simulink model "LLC_Resonant_Converter_v1"  (R2024b)
settings: Solver=FixedStepDiscrete  StartTime=0.0  StopTime=0.3  FixedStep=Ts_Power  MaxStep=1e-7  RelTol=1e-4  EnableMultiTasking=on
PreLoadFcn:
  | LLC_Resonant_Converter_v1_data
values from neighbouring files (symbols this model uses):
  Co = 150e-6    (= 0.00015)    [LLC_Resonant_Converter_v1_data.m]    (also in OBC_v1_data.m)
  Cr = 75e-9    (= 7.5e-08)    [LLC_Resonant_Converter_v1_data.m]    (also in OBC_v1_data.m)
  fs_LCC_max = 250e3    (= 250000)    [LLC_Resonant_Converter_v1_data.m]    (also in OBC_v1_data.m = 300000)
  fs_LCC_min = 120e3    (= 120000)    [LLC_Resonant_Converter_v1_data.m]    (also in OBC_v1_data.m)
  Ki_LLC = 150e3    (= 150000)    [LLC_Resonant_Converter_v1_data.m]    (also in OBC_v1_data.m)
  Kp_LLC = 100    [LLC_Resonant_Converter_v1_data.m]    (also in OBC_v1_data.m = 25)
  Lm = 150e-6    (= 0.00015)    [LLC_Resonant_Converter_v1_data.m]    (also in OBC_v1_data.m)
  Lr = 25e-6    (= 2.5e-05)    [LLC_Resonant_Converter_v1_data.m]    (also in OBC_v1_data.m)
  Np = 10    [LLC_Resonant_Converter_v1_data.m]    (also in OBC_v1_data.m)
  Ns = 12    [LLC_Resonant_Converter_v1_data.m]    (also in OBC_v1_data.m)
  Po_nom = 7.2e3    (= 7200)    [LLC_Resonant_Converter_v1_data.m]    (also in OBC_v1_data.m)
  Ts_Control = 10e-6    (= 1e-05)    [LLC_Resonant_Converter_v1_data.m]    (also in OBC_v1_data.m; Totem_Pole_PFC_v1_data.m)
  Ts_Power = 50e-9    (= 5e-08)    [LLC_Resonant_Converter_v1_data.m]    (also in OBC_v1_data.m; Totem_Pole_PFC_v1_data.m)
  Vdc_in = 400    [LLC_Resonant_Converter_v1_data.m]    (also in OBC_v1_data.m)
  Vo_nom = 400    [LLC_Resonant_Converter_v1_data.m]    (also in OBC_v1_data.m)
undefined symbols (not defined in the file or in its folder): DiscIntNeverNeededParam
libraries: spsSeriesRLCBranchLib x5, spsDiodeLib x4, MyLibrary x4, spsMeanLib x3, spsCurrentMeasurementLib x3, spsVoltageMeasurementLib x3, spsOnDelayLib x2, spsDCVoltageSourceLib x1, spsIdealSwitchLib x1, spsLinearTransformerLib x1, spspowerguiLib x1
settings Model: SimulationMode=accelerator  Creator=The MathWorks, Inc.  LastModifiedBy=santh
settings SolverCC: AlgebraicLoopSolver=TrustRegion  SolverResetMethod=Robust
settings DataIOCC: SaveOutput=off  SignalLogging=off  DSMLogging=off  SaveTime=off  ReturnWorkspaceOutputs=off
settings OptimizationCC: LifeSpan=inf
settings DebuggingCC: UnconnectedInputMsg=warning  UnconnectedOutputMsg=warning  UnconnectedLineMsg=warning  SFUnexpectedBacktrackingDiag=warning  SFNoUnconditionalDefaultTransitionDiag=warning  SFExecutionAtInitializationDiag=none  ArithmeticOperatorsInVariantConditions=warning
settings ModelReferenceCC: EnableRefExpFcnMdlSchedulingChecks=on
settings SFSimCC: SimUseLocalCustomCode=off  CustomCodeUndefinedFunction=UseInterfaceOnly
settings RTWCC: RTWUseLocalCustomCode=off  GPUComputeCapability=3.5  DLArmComputeVersion=19.05
settings CodeAppCC: StateflowObjectComments=on
settings GRTTargetCC: TargetLangStandard=C89/C90 (ANSI)
settings ConfigComp: CovMetricSettings=dw  CovSaveCumulativeToWorkspaceVar=on  CovSaveSingleToWorkspaceVar=on  CovExternalEMLEnable=off
settings SimscapeCC: SimscapeNormalizeSystem=off  SimscapeNominalValues={1, 'bar'; 1, 'cm^3/s'; 1, 'bar*kg/s'; 1, 'kJ/kg'; 1, 'kW'; }

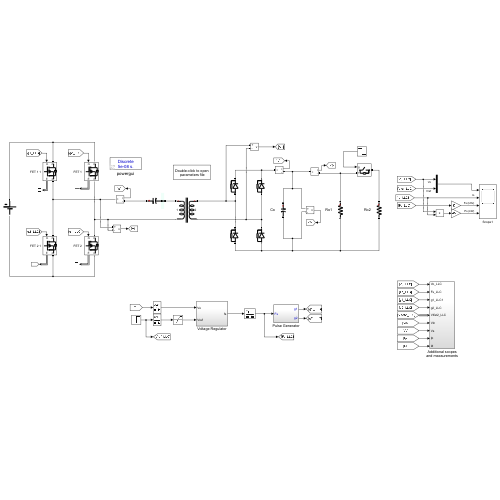
[thumbnail: Simulink's stored preview of the top-level diagram]
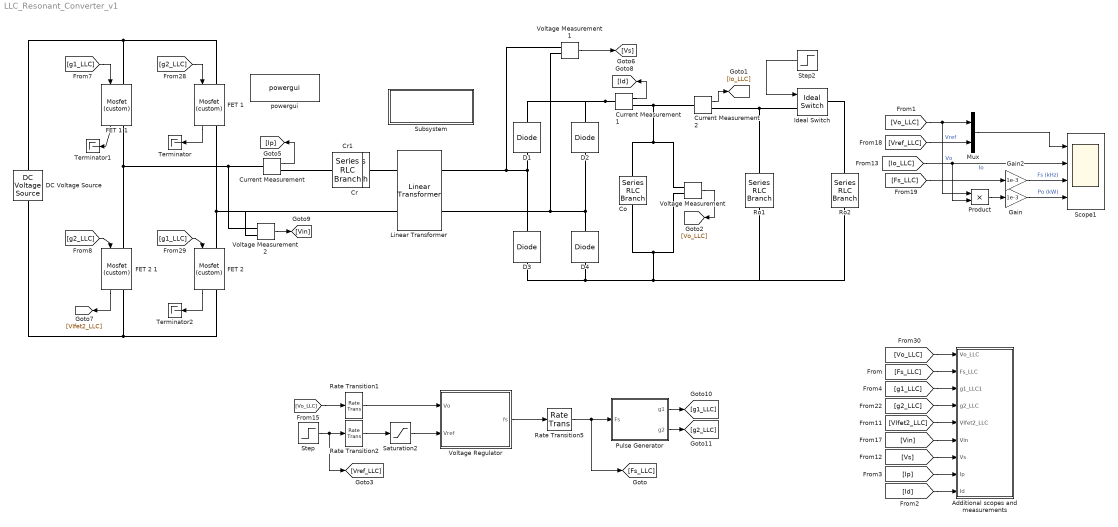
== system LLC_Resonant_Converter_v1 ==
  Additional scopes and measurements : Subsystem
  Co : spsSeriesRLCBranchLib/Series RLC Branch  LConnTagsString=__new0  RConnTagsString=__new0  BranchType=C  Resistance=1e-4  Inductance=200e-6  SetiL0=off  InitialCurrent=0  Capacitance=Co  Setx0=on  InitialVoltage=350  Measurements=None
  Cr : spsSeriesRLCBranchLib/Series RLC Branch  LConnTagsString=__new0  RConnTagsString=__new0  BranchType=C  Resistance=1e-4  Inductance=200e-6  SetiL0=off  InitialCurrent=0  Capacitance=Cr  Setx0=off  InitialVoltage=40  Measurements=None
  Cr1 : spsSeriesRLCBranchLib/Series RLC Branch  LConnTagsString=__new0  RConnTagsString=__new0  BranchType=C  Resistance=1e-4  Inductance=200e-6  SetiL0=off  InitialCurrent=0  Capacitance=Cr  Setx0=off  InitialVoltage=40  Measurements=None
  Current Measurement : spsCurrentMeasurementLib/Current Measurement  PhasorSimulation=off  OutputType=Complex  PSBequivalent=0
  Current Measurement1 : spsCurrentMeasurementLib/Current Measurement  PhasorSimulation=off  OutputType=Complex  PSBequivalent=0
  Current Measurement2 : spsCurrentMeasurementLib/Current Measurement  PhasorSimulation=off  OutputType=Complex  PSBequivalent=0
  D{1..4} (4 alike) : spsDiodeLib/Diode  Ron=Ron_Diode  Lon=0  Vf=Vf  IC=0  UseSnubber=off  Rs=1e6  Cs=inf  Measurements=off
  DC Voltage Source : spsDCVoltageSourceLib/DC Voltage Source  Amplitude=Vdc_in  Measurements=None
  "FET 1 " : MyLibrary/Mosfet (custom)  Ron=Ron_FET  Lon=0  Rd=Ron_Diode  Vfd=Vf  IC=0  Rs=1e6  Cs=inf  Measurements=on
  FET 1 1 : MyLibrary/Mosfet (custom)  Ron=Ron_FET  Lon=0  Rd=Ron_Diode  Vfd=Vf  IC=0  Rs=1e6  Cs=inf  Measurements=on
  "FET 2 " : MyLibrary/Mosfet (custom)  Ron=Ron_FET  Lon=0  Rd=Ron_Diode  Vfd=Vf  IC=0  Rs=1e6  Cs=inf  Measurements=on
  FET 2 1 : MyLibrary/Mosfet (custom)  Ron=Ron_FET  Lon=0  Rd=Ron_Diode  Vfd=Vf  IC=0  Rs=1e6  Cs=inf  Measurements=on
  Gain : Gain  Gain=1e-3
  Gain2 : Gain  Gain=1e-3
  Ideal Switch : spsIdealSwitchLib/Ideal Switch  Ron=0.001  Lon=0  IC=1  Rs=1e5  Cs=inf  Measurements=off
  Linear Transformer : spsLinearTransformerLib/Linear Transformer  UNITS=SI  NominalPower=[ 7000 100e3 ]  winding1="[Np   1e-2 Lr]"  winding2="[Ns  1e-2  1e-8 ]"  ThreeWindings=off  winding3=[3.15e+05 0.7938 0.084225]  RmLm=[1e4 Lm]  Measurements=None  DataType=on
  Mux : Mux  Inputs=2
  Product : Product
  Pulse Generator : Subsystem
  Rate Transition1 : RateTransition  OutPortSampleTime=Ts_Control
  Rate Transition2 : RateTransition  OutPortSampleTime=Ts_Control
  Rate Transition5 : RateTransition  InitialCondition=fs_LCC_min  OutPortSampleTime=Ts_Power
  Ro1 : spsSeriesRLCBranchLib/Series RLC Branch  LConnTagsString=__new0  RConnTagsString=__new0  BranchType=R  Resistance=Vo_nom^2/(0.1*Po_nom)  Inductance=200e-6  SetiL0=off  InitialCurrent=0  Capacitance=400e-6  Setx0=off  InitialVoltage=0  Measurements=None
  Ro2 : spsSeriesRLCBranchLib/Series RLC Branch  LConnTagsString=__new0  RConnTagsString=__new0  BranchType=R  Resistance=Vo_nom^2/(0.9*Po_nom)  Inductance=200e-6  SetiL0=off  InitialCurrent=0  Capacitance=400e-6  Setx0=off  InitialVoltage=0  Measurements=None
  Saturation2 : Saturate  UpperLimit=450  LowerLimit=275
  Scope1 : Scope  NumInputPorts=4
  Step : Step  Time=0.1  Before=350  After=400  SampleTime=Ts_Power
  Step2 : Step  Time=0.2  Before=1  After=0  SampleTime=Ts_Power
  Subsystem : Subsystem
      settings: OpenFcn=edit('LLC_Resonant_Converter_v1_data');
      mask Display: disp('Double-click to open\n parameters file');
  Terminator : Terminator
  Terminator1 : Terminator
  Terminator2 : Terminator
  Voltage Measurement : spsVoltageMeasurementLib/Voltage Measurement  PhasorSimulation=off  OutputType=Complex  PSBequivalent=0
  Voltage Measurement1 : spsVoltageMeasurementLib/Voltage Measurement  PhasorSimulation=off  OutputType=Complex  PSBequivalent=0
  Voltage Measurement2 : spsVoltageMeasurementLib/Voltage Measurement  PhasorSimulation=off  OutputType=Complex  PSBequivalent=0
  Voltage Regulator : Subsystem
  powergui : spspowerguiLib/powergui  Priority=1  SimulationMode=Discrete  SampleTime=Ts_Power  frequency=60  Iterations=50  frequencyindice=0  Pbase=100e6  ErrMax=1e-4  UnitsV=kV  UnitsW=MW  buscounter=0  FunctionMessages=off  echomessages=off  EnableUseOfTLC=off  CurrentSourceSwitches=off  DisableSnubberDevices=off  DisableRonSwitches=off  DisableVfSwitches=off  DisplayEquations=off  AutomaticDiscreteSolvers=off  SolverType=Tustin/Backward Euler (TBE)  Interpol=off  ExternalGateDelay=off  methode=off  Ts=100  x0status=blocks  SPID=on  SwTol=0  HookPort=off  NonlinearTolerance=1e-4  nMaxIteration=100  ContinueOnMaxIteration=off  RestoreLinks=warning  ResistiveCurrentMeasurement=off  Frange=[0:2:500]  Ylog=off  Xlog=on  ShowGrid=off  save=off  variable=ZData  structure=0  ZoomFFT=off  StartTime=0.0  cycles=1  DisplayStyle=1  fundamental=60  FreqAxis=off  MaxFrequency=1000  frequencyindicesteady=1  RmsSteady=1  display=off
  wires:
  [g1_LLC] -> "FET 2 "/1
  Current Measurement/1 -> [Ip]
  Voltage Measurement/1 -> [Vo_LLC]
  Current Measurement1/1 -> [Id]
  [Vo_LLC] -> Rate Transition1/1
  Pulse Generator/1(g1) -> [g1_LLC]
  Pulse Generator/2(g2) -> [g2_LLC]
  Current Measurement2/1 -> [Io_LLC]
  "FET 1 "/1 -> Terminator/1
  Rate Transition2/1 -> Saturation2/1
  Saturation2/1 -> Voltage Regulator/2(Vref)
  Step/1 -> [Vref_LLC], Rate Transition2/1
  Rate Transition1/1 -> Voltage Regulator/1(Vo)
  Step2/1 -> Ideal Switch/1
  [g2_LLC] -> "FET 1 "/1
  "FET 2 "/1 -> Terminator2/1
  Gain2/1 -> Scope1/3  "Fs (kHz)"
  [Vref_LLC] -> Mux/2  "Vref"
  Product/1 -> Gain/1
  [Io_LLC] -> Product/2, Scope1/2  "Io"
  [Vo_LLC] -> Product/1, Mux/1  "Vo"
  [Fs_LLC] -> Gain2/1
  Gain/1 -> Scope1/4  "Po (kW)"
  Voltage Measurement1/1 -> [Vs]
  Voltage Measurement2/1 -> [Vin]
  Rate Transition5/1 -> [Fs_LLC], Pulse Generator/1(Fs)
  FET 2 1/1 -> [VIfet2_LLC]
  [g1_LLC] -> FET 1 1/1
  FET 1 1/1 -> Terminator1/1
  [g2_LLC] -> FET 2 1/1
  Voltage Regulator/1(fs) -> Rate Transition5/1
  [Vo_LLC] -> Additional scopes and measurements/1(Vo_LLC)
  [Fs_LLC] -> Additional scopes and measurements/2(Fs_LLC)
  [g2_LLC] -> Additional scopes and measurements/4(g2_LLC)
  [Vs] -> Additional scopes and measurements/7(Vs)
  [Vin] -> Additional scopes and measurements/6(Vin)
  [Id] -> Additional scopes and measurements/9(Id)
  [Ip] -> Additional scopes and measurements/8(Ip)
  Mux/1 -> Scope1/1
  [g1_LLC] -> Additional scopes and measurements/3(g1_LLC1)
  [VIfet2_LLC] -> Additional scopes and measurements/5(VIfet2_LLC)
  connections:
  Co/RConn1 -- Voltage Measurement/LConn2 -- Ro2/RConn1 -- Ro1/RConn1 -- D3/LConn1 -- D4/LConn1
  Linear Transformer/RConn1 -- D3/RConn1 -- D1/LConn1 -- Voltage Measurement1/LConn1
  Linear Transformer/RConn2 -- Voltage Measurement1/LConn2 -- D2/LConn1 -- D4/RConn1
  Cr/LConn1 -- Current Measurement/RConn1
  Linear Transformer/LConn1 -- Cr/RConn1
  Current Measurement1/LConn1 -- D1/RConn1 -- D2/RConn1
  Voltage Measurement/LConn1 -- Current Measurement2/LConn1 -- Current Measurement1/RConn1 -- Co/LConn1
  Current Measurement2/RConn1 -- Ideal Switch/LConn1 -- Ro1/LConn1
  DC Voltage Source/LConn1 -- "FET 2 "/RConn1 -- FET 2 1/RConn1
  Ro2/LConn1 -- Ideal Switch/RConn1
  DC Voltage Source/RConn1 -- FET 1 1/LConn1 -- "FET 1 "/LConn1
  Voltage Measurement2/LConn1 -- Current Measurement/LConn1 -- FET 1 1/RConn1 -- FET 2 1/LConn1
  "FET 1 "/RConn1 -- "FET 2 "/LConn1 -- Linear Transformer/LConn2 -- Voltage Measurement2/LConn2

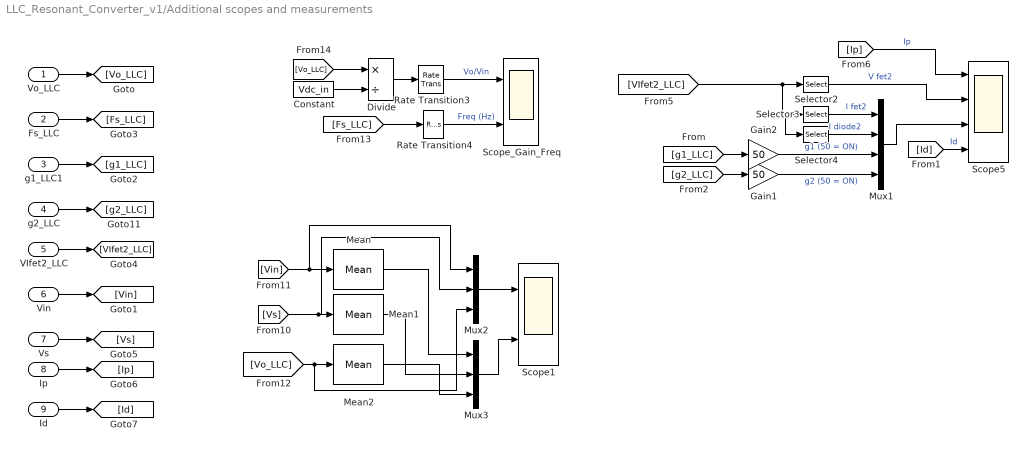
== system LLC_Resonant_Converter_v1/Additional scopes and measurements ==
  Vo_LLC : Inport
  Fs_LLC : Inport  Port=2
  g1_LLC1 : Inport  Port=3
  g2_LLC : Inport  Port=4
  VIfet2_LLC : Inport  Port=5
  Vin : Inport  Port=6
  Vs : Inport  Port=7
  Ip : Inport  Port=8
  Id : Inport  Port=9
  Constant : Constant  Value=Vdc_in
  Divide : Product  Inputs=*/
  Gain1 : Gain  Gain=50
  Gain2 : Gain  Gain=50
  Mean : spsMeanLib/Mean  Freq=150e3  Vinit=0  Ts=Ts_Power
  Mean1 : spsMeanLib/Mean  Freq=150e3  Vinit=0  Ts=Ts_Power
  Mean2 : spsMeanLib/Mean  Freq=150e3  Vinit=0  Ts=Ts_Power
  Mux1 : Mux
  Mux2 : Mux  Inputs=3
  Mux3 : Mux  Inputs=3
  Rate Transition3 : RateTransition  OutPortSampleTime=Ts_Power*100
  Rate Transition4 : RateTransition  OutPortSampleTime=Ts_Power*100
  Scope1 : Scope  NumInputPorts=2
  Scope5 : Scope  NumInputPorts=4
  Scope_Gain_Freq : Scope  NumInputPorts=2
  Selector2 : Selector  InputPortWidth=3  IndexOptions=Index vector (dialog)  Indices=2  OutputSizes=1
  Selector3 : Selector  InputPortWidth=3  IndexOptions=Index vector (dialog)  Indices=1  OutputSizes=1
  Selector4 : Selector  InputPortWidth=3  IndexOptions=Index vector (dialog)  Indices=3  OutputSizes=1
  wires:
  [VIfet2_LLC] -> Selector4/1, Selector3/1, Selector2/1
  Selector2/1 -> Scope5/2  "V fet2"
  Mux1/1 -> Scope5/3
  [Ip] -> Scope5/1  "Ip"
  Selector4/1 -> Mux1/2  "I diode2"
  Selector3/1 -> Mux1/1  "I fet2"
  [Id] -> Scope5/4  "Id"
  Vo_LLC/1 -> [Vo_LLC]
  Fs_LLC/1 -> [Fs_LLC]
  VIfet2_LLC/1 -> [VIfet2_LLC]
  g2_LLC/1 -> [g2_LLC]
  [g2_LLC] -> Gain1/1
  Vs/1 -> [Vs]
  Vin/1 -> [Vin]
  [Vo_LLC] -> Mux2/3, Mean2/1
  Mean2/1 -> Mux3/3
  Mean1/1 -> Mux3/2
  Mux2/1 -> Scope1/1
  Mean/1 -> Mux3/1
  [Vs] -> Mux2/2, Mean1/1
  Mux3/1 -> Scope1/2
  [Vin] -> Mux2/1, Mean/1
  Rate Transition3/1 -> Scope_Gain_Freq/1  "Vo/Vin"
  [Vo_LLC] -> Divide/1
  Divide/1 -> Rate Transition3/1
  Constant/1 -> Divide/2
  Rate Transition4/1 -> Scope_Gain_Freq/2  "Freq (Hz)"
  [Fs_LLC] -> Rate Transition4/1
  Ip/1 -> [Ip]
  Id/1 -> [Id]
  g1_LLC1/1 -> [g1_LLC]
  Gain1/1 -> Mux1/4  "g2 (50 = ON)"
  [g1_LLC] -> Gain2/1
  Gain2/1 -> Mux1/3  "g1 (50 = ON)"

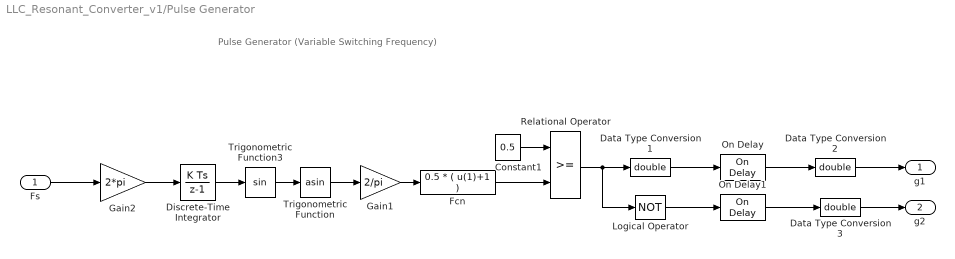
== system LLC_Resonant_Converter_v1/Pulse Generator ==
  note: Pulse Generator
      | (Variable Switching Frequency)
  Fs : Inport
  Constant1 : Constant  Value=0.5
  Data Type Conversion1 : DataTypeConversion  OutDataTypeStr=double  SaturateOnIntegerOverflow=off  RndMeth=Floor
  Data Type Conversion2 : DataTypeConversion  OutDataTypeStr=double  SaturateOnIntegerOverflow=off  RndMeth=Floor
  Data Type Conversion3 : DataTypeConversion  OutDataTypeStr=double  SaturateOnIntegerOverflow=off  RndMeth=Floor
  Discrete-Time Integrator : DiscreteIntegrator  SampleTime=Ts_Power  ICPrevOutput=DiscIntNeverNeededParam  ICPrevScaledInput=DiscIntNeverNeededParam
  Fcn : Fcn  Expr=0.5 * ( u(1)+1 )
  Gain1 : Gain  Gain=2/pi  SaturateOnIntegerOverflow=on  OutDataTypeStr=Inherit: Same as input  ParamDataTypeStr=Inherit: Same as input
  Gain2 : Gain  Gain=2*pi  SaturateOnIntegerOverflow=on  OutDataTypeStr=Inherit: Same as input  ParamDataTypeStr=Inherit: Same as input
  Logical Operator : Logic  Operator=NOT  AllPortsSameDT=off  OutDataTypeStr=float('double')
  On Delay : spsOnDelayLib/On Delay  DelayType=On delay  delay=DT_LLC  ic=0  Ts=Ts_Power
  On Delay1 : spsOnDelayLib/On Delay  DelayType=On delay  delay=DT_LLC  ic=0  Ts=Ts_Power
  Relational Operator : RelationalOperator  OutDataTypeStr=boolean  InputSameDT=off
  Trigonometric Function : Trigonometry  Operator=asin
  Trigonometric Function3 : Trigonometry
  g1 : Outport  VectorParamsAs1DForOutWhenUnconnected=off
  g2 : Outport  Port=2  VectorParamsAs1DForOutWhenUnconnected=off
  wires:
  On Delay1/1 -> Data Type Conversion3/1
  On Delay/1 -> Data Type Conversion2/1
  Fs/1 -> Gain2/1
  Gain2/1 -> Discrete-Time Integrator/1
  Data Type Conversion1/1 -> On Delay/1
  Logical Operator/1 -> On Delay1/1
  Fcn/1 -> Relational Operator/2
  Relational Operator/1 -> Logical Operator/1, Data Type Conversion1/1
  Constant1/1 -> Relational Operator/1
  Discrete-Time Integrator/1 -> Trigonometric Function3/1
  Trigonometric Function/1 -> Gain1/1
  Gain1/1 -> Fcn/1
  Trigonometric Function3/1 -> Trigonometric Function/1
  Data Type Conversion2/1 -> g1/1
  Data Type Conversion3/1 -> g2/1

== system LLC_Resonant_Converter_v1/Subsystem ==

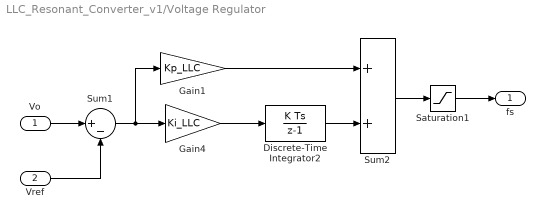
== system LLC_Resonant_Converter_v1/Voltage Regulator ==
  Vo : Inport
  Vref : Inport  Port=2
  Discrete-Time Integrator2 : DiscreteIntegrator  InitialCondition=fs_LCC_min  SampleTime=Ts_Control  LimitOutput=on  UpperSaturationLimit=fs_LCC_max  LowerSaturationLimit=fs_LCC_min  ICPrevOutput=DiscIntNeverNeededParam  ICPrevScaledInput=DiscIntNeverNeededParam
  Gain1 : Gain  Gain=Kp_LLC  SaturateOnIntegerOverflow=on  OutDataTypeStr=Inherit: Same as input  ParamDataTypeStr=Inherit: Same as input
  Gain4 : Gain  Gain=Ki_LLC  SaturateOnIntegerOverflow=on  OutDataTypeStr=Inherit: Same as input  ParamDataTypeStr=Inherit: Same as input
  Saturation1 : Saturate  UpperLimit=fs_LCC_max  LowerLimit=fs_LCC_min
  Sum1 : Sum  Inputs=|+-  InputSameDT=on  SaturateOnIntegerOverflow=on  OutDataTypeStr=Inherit: Same as first input
  Sum2 : Sum  InputSameDT=on  SaturateOnIntegerOverflow=on  OutDataTypeStr=Inherit: Same as first input
  fs : Outport  VectorParamsAs1DForOutWhenUnconnected=off
  wires:
  Saturation1/1 -> fs/1
  Gain1/1 -> Sum2/1
  Sum2/1 -> Saturation1/1
  Discrete-Time Integrator2/1 -> Sum2/2
  Gain4/1 -> Discrete-Time Integrator2/1
  Sum1/1 -> Gain4/1, Gain1/1
  Vo/1 -> Sum1/1
  Vref/1 -> Sum1/2
